simulink model "vsi_spwm"  (R2018a)
settings: Solver=FixedStepDiscrete  StartTime=0.0  StopTime=2/cfg.fl  FixedStep=cfg.fpga.ts  RelTol=1e-3
PreLoadFcn:
  | vsi_spwm_config;
InitFcn:
  | vsi_spwm_config;
undefined symbols (not defined in the file or in its folder): cfg
libraries: powerlib x18, hdlsllib x11, simulink x2
settings Model: DataTypeOverride=Off  Creator=CIDEI  LastModifiedBy=pcoss
settings DataIOCC: SaveOutput=off  SaveTime=off
settings OptimizationCC: BlockReduction=off  ConditionallyExecuteInputs=off  DefaultParameterBehavior=Inlined  LifeSpan=inf
settings DebuggingCC: AlgebraicLoopMsg=error  SingleTaskRateTransMsg=error  StrictBusMsg=ErrorOnBusTreatedAsVector  SFUnexpectedBacktrackingDiag=warning  SFNoUnconditionalDefaultTransitionDiag=warning  SFExecutionAtInitializationDiag=none
settings HardwareCC: ProdBitPerPointer=32  ProdBitPerSizeT=32  ProdBitPerPtrDiffT=32  ProdLargestAtomicFloat=None  ProdIntDivRoundTo=Undefined  ProdEndianess=Unspecified  ProdWordSize=32  ProdHWDeviceType=ASIC/FPGA->ASIC/FPGA  ProdEqTarget=off
settings CodeAppCC: StateflowObjectComments=on
settings GRTTargetCC: TargetLangStandard=C89/C90 (ANSI)
settings ConfigComp: CovMetricSettings=dw  CovHtmlReporting=on  CovSaveCumulativeToWorkspaceVar=on  CovSaveSingleToWorkspaceVar=on  CovExternalEMLEnable=off
settings SimscapeCC: SimscapeNormalizeSystem=off

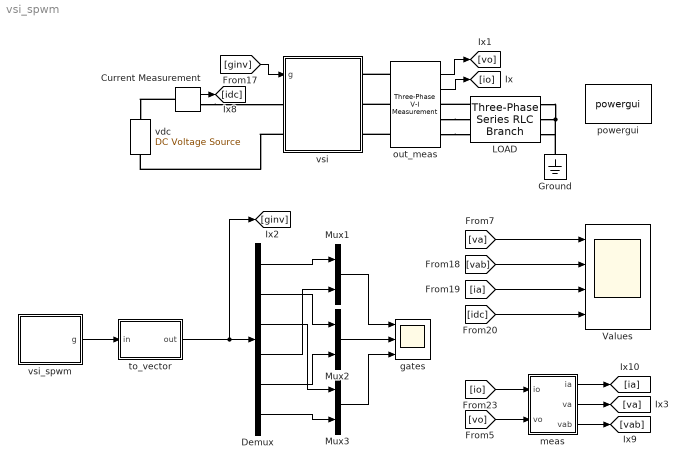
== system vsi_spwm ==
  Current Measurement : powerlib/Measurements/Current Measurement  PhasorSimulation=off  OutputType=Complex  PSBequivalent=0
  Demux : Demux  Outputs=6
  Ground : powerlib/Elements/Ground  LConnTagsString=a
  LOAD : powerlib/Elements/Three-Phase Series RLC Branch  LConnTagsString=A|B|C  RConnTagsString=A|B|C  BranchType=RL  Resistance=cfg.r  Inductance=cfg.l  Capacitance=1e-6  Measurements=None
  Mux1 : Mux  Inputs=2
  Mux2 : Mux  Inputs=2
  Mux3 : Mux  Inputs=2
  Values : Scope  NumInputPorts=4
  gates : Scope  NumInputPorts=3
  meas : Subsystem
  out_meas : powerlib/Measurements/Three-Phase V-I Measurement  VoltageMeasurement=phase-to-ground  SetLabelV=off  LabelV=Vabc  Vpu=off  VpuLL=off  CurrentMeasurement=yes  SetLabelI=off  LabelI=Iabc  Ipu=off  Pbase=100e6  Vbase=500e3  OutputType=Complex  PhasorSimulation=off  PSBequivalent=0
  powergui : powerlib/powergui  Priority=1  SimulationMode=Discrete  SampleTime=cfg.ts  frequency=60  Iterations=50  frequencyindice=0  Pbase=100e6  ErrMax=1e-4  UnitsV=kV  UnitsW=MW  buscounter=0  FunctionMessages=off  echomessages=off  EnableUseOfTLC=off  CurrentSourceSwitches=off  DisableSnubberDevices=off  DisableRonSwitches=off  DisableVfSwitches=off  DisplayEquations=off  SolverType=Backward Euler  Interpol=off  ExternalGateDelay=off  methode=off  Ts=0  x0status=blocks  SPID=off  SwTol=0  HookPort=off  RestoreLinks=warning  ResistiveCurrentMeasurement=off  Frange=[0:2:500]  Ylog=off  Xlog=on  ShowGrid=off  save=off  variable=ZData  structure=one_mod_model  ZoomFFT=off  StartTime=0.12  cycles=1  DisplayStyle=1  fundamental=50  FreqAxis=off  MaxFrequency=1000  frequencyindicesteady=1  RmsSteady=1  display=off
  to_vector : Subsystem
  vdc : powerlib/Electrical Sources/DC Voltage Source  Amplitude=cfg.vdc  Measurements=None
  vsi : Subsystem
  vsi_spwm : Subsystem
  wires:
  Mux2/1 -> gates/2
  Mux1/1 -> gates/1
  Mux3/1 -> gates/3
  Demux/4 -> Mux1/2
  Demux/5 -> Mux2/2
  Demux/6 -> Mux3/2
  out_meas/2 -> [io]
  out_meas/1 -> [vo]
  Current Measurement/1 -> [idc]
  [ginv] -> vsi/1(g)
  vsi_spwm/1(g) -> to_vector/1(in)
  Demux/1 -> Mux1/1
  Demux/2 -> Mux2/1
  Demux/3 -> Mux3/1
  [vab] -> Values/2
  [ia] -> Values/3
  [idc] -> Values/4
  [va] -> Values/1
  [io] -> meas/1(io)
  [vo] -> meas/2(vo)
  meas/1(ia) -> [ia]
  meas/3(vab) -> [vab]
  to_vector/1(out) -> [ginv], Demux/1
  meas/2(va) -> [va]
  connections:
  LOAD/RConn2 -- LOAD/RConn1 -- Ground/LConn1 -- LOAD/RConn3
  LOAD/LConn1 -- out_meas/RConn1
  Current Measurement/RConn1 -- vsi/LConn1
  out_meas/LConn2 -- vsi/RConn2
  out_meas/RConn3 -- LOAD/LConn3
  out_meas/RConn2 -- LOAD/LConn2
  out_meas/LConn1 -- vsi/RConn1
  out_meas/LConn3 -- vsi/RConn3
  Current Measurement/LConn1 -- vdc/RConn1
  vsi/LConn2 -- vdc/LConn1

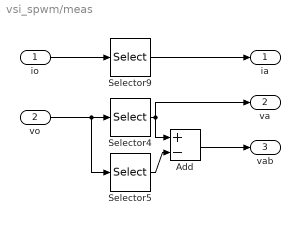
== system vsi_spwm/meas ==
  io : Inport
  vo : Inport  Port=2
  Add : Sum  Inputs=+-
  Selector4 : Selector  InputPortWidth=3  IndexOptions=Index vector (dialog)  Indices=1  OutputSizes=1
  Selector5 : Selector  InputPortWidth=3  IndexOptions=Index vector (dialog)  Indices=2  OutputSizes=1
  Selector9 : Selector  InputPortWidth=3  IndexOptions=Index vector (dialog)  Indices=1  OutputSizes=1
  ia : Outport
  va : Outport  Port=2
  vab : Outport  Port=3
  wires:
  vo/1 -> Selector5/1, Selector4/1
  Selector4/1 -> va/1, Add/1
  Selector5/1 -> Add/2
  Add/1 -> vab/1
  Selector9/1 -> ia/1
  io/1 -> Selector9/1

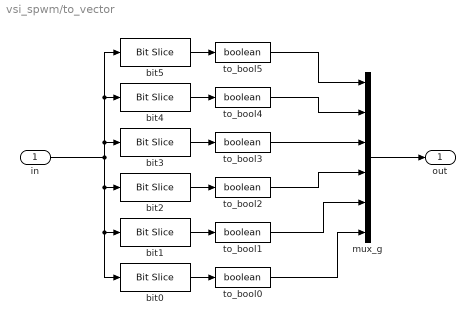
== system vsi_spwm/to_vector ==
  in : Inport
  bit0 : hdlsllib/Logic and Bit Operations/Bit Slice  lidx=0  ridx=0
  bit1 : hdlsllib/Logic and Bit Operations/Bit Slice  lidx=1  ridx=1
  bit2 : hdlsllib/Logic and Bit Operations/Bit Slice  lidx=2  ridx=2
  bit3 : hdlsllib/Logic and Bit Operations/Bit Slice  lidx=3  ridx=3
  bit4 : hdlsllib/Logic and Bit Operations/Bit Slice  lidx=4  ridx=4
  bit5 : hdlsllib/Logic and Bit Operations/Bit Slice  lidx=5  ridx=5
  mux_g : Mux  Inputs=6
  to_bool{0..5} (6 alike) : DataTypeConversion  OutDataTypeStr=boolean
  out : Outport
  wires:
  to_bool0/1 -> mux_g/6
  to_bool2/1 -> mux_g/4
  to_bool3/1 -> mux_g/3
  bit4/1 -> to_bool4/1
  bit5/1 -> to_bool5/1
  bit3/1 -> to_bool3/1
  bit2/1 -> to_bool2/1
  mux_g/1 -> out/1
  to_bool5/1 -> mux_g/1
  to_bool4/1 -> mux_g/2
  bit1/1 -> to_bool1/1
  to_bool1/1 -> mux_g/5
  in/1 -> bit5/1, bit4/1, bit3/1, bit2/1, bit1/1, bit0/1
  bit0/1 -> to_bool0/1

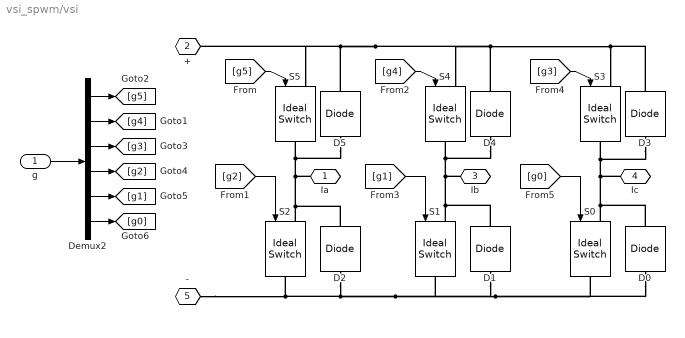
== system vsi_spwm/vsi ==
  g : Inport
  D{0..5} (6 alike) : powerlib/Power Electronics/Diode  Ron=cfg.diode.Ron  Lon=0  Vf=0  IC=0  UseSnubber=off  Rs=cfg.diode.snubber_Rs  Cs=cfg.diode.snubber_Cs  Measurements=off
  Demux2 : Demux  Outputs=6
  S{0..5} (6 alike) : powerlib/Power Electronics/Ideal Switch  Ron=cfg.switch.Ron  Lon=0  IC=0  Rs=cfg.switch.snubber_Rs  Cs=cfg.switch.snubber_Cs  Measurements=off
  Ia : PMIOPort  Side=Right
  + : PMIOPort  Port=2  Side=Left
  Ib : PMIOPort  Port=3  Side=Right
  Ic : PMIOPort  Port=4  Side=Right
  - : PMIOPort  Port=5  Side=Left
  wires:
  Demux2/1 -> [g5]
  Demux2/4 -> [g2]
  g/1 -> Demux2/1
  [g2] -> S2/1
  [g4] -> S4/1
  [g1] -> S1/1
  Demux2/5 -> [g1]
  [g3] -> S3/1
  [g0] -> S0/1
  Demux2/6 -> [g0]
  Demux2/3 -> [g3]
  Demux2/2 -> [g4]
  [g5] -> S5/1
  connections:
  S2/LConn1 -- D2/RConn1 -- D5/LConn1 -- S5/RConn1 -- Ia/RConn1
  S1/LConn1 -- D1/RConn1 -- D4/LConn1 -- S4/RConn1 -- Ib/RConn1
  S0/LConn1 -- D0/RConn1 -- D3/LConn1 -- S3/RConn1 -- Ic/RConn1
  S4/LConn1 -- D5/RConn1 -- S5/LConn1 -- +/RConn1 -- D3/RConn1 -- S3/LConn1 -- D4/RConn1
  -/RConn1 -- D1/LConn1 -- D0/LConn1 -- S0/RConn1 -- S1/RConn1 -- D2/LConn1 -- S2/RConn1

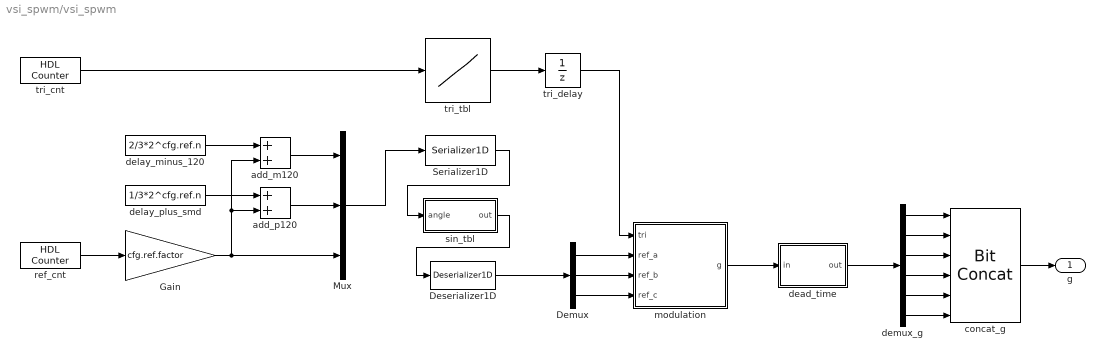
== system vsi_spwm/vsi_spwm ==
  Demux : Demux  Outputs=3
  Deserializer1D : hdlsllib/HDL Operations/Deserializer1D  Ratio=3  IdleCycles=0  InitialCondition=0  startIn=off  validIn=off  validOut=off  inputDataDimensions=-1  inputSampleTime=-1  inputSignalType=auto
      settings: SourceProductName=HDL Coder  SourceProductBaseCode=HD
  Gain : Gain  Gain=cfg.ref.factor  OutDataTypeStr=fixdt(0,cfg.ref.n,0)
  Mux : Mux  Inputs=3
  Serializer1D : hdlsllib/HDL Operations/Serializer1D  Ratio=3  IdleCycles=0  validIn=off  startOut=off  validOut=off  inputDataDimensions=-1  inputSampleTime=-1  inputSignalType=auto
      settings: SourceProductName=HDL Coder  SourceProductBaseCode=HD
  add_m120 : Sum  OutDataTypeStr=Inherit: Same as accumulator
  add_p120 : Sum  OutDataTypeStr=Inherit: Same as accumulator
  concat_g : hdlsllib/Logic and Bit Operations/Bit Concat  numInputs=6
      settings: SourceProductName=HDL Coder  SourceProductBaseCode=HD
  dead_time : Subsystem
  delay_minus_120 : Constant  Value=2/3*2^cfg.ref.n  OutDataTypeStr=fixdt(0,cfg.ref.n,0)  SampleTime=-1
  delay_plus_smd : Constant  Value=1/3*2^cfg.ref.n  OutDataTypeStr=fixdt(0,cfg.ref.n,0)  SampleTime=-1
  demux_g : Demux  Outputs=6
  modulation : Subsystem
  ref_cnt : hdlsllib/Sources/HDL Counter  CountType=Count limited  CountInit=0  CountStep=1  CountMax=1/cfg.fl/cfg.ts  CountFromType=Initial value  CountFrom=0  CountResetPort=off  CountLoadPort=off  CountEnbPort=off  CountDirPort=off  CountDataType=Unsigned  CountWordLen=ceil(log2(1/cfg.fl/cfg.ts))  CountFracLen=0  CountSampTime=cfg.ts
      settings: SourceProductBaseCode=HD
  sin_tbl : Subsystem
  tri_cnt : hdlsllib/Sources/HDL Counter  CountType=Count limited  CountInit=0  CountStep=1  CountMax=length(cfg.tri.data)-1  CountFromType=Initial value  CountFrom=0  CountResetPort=off  CountLoadPort=off  CountEnbPort=off  CountDirPort=off  CountDataType=Unsigned  CountWordLen=cfg.tri.n  CountFracLen=0  CountSampTime=cfg.ts
      settings: SourceProductBaseCode=HD
  tri_delay : UnitDelay  SampleTime=-1
  tri_tbl : Lookup_n-D  NumberOfTableDimensions=1  BreakpointsForDimension1=[0:length(cfg.tri.data)-1]  BreakpointsForDimension1FirstPoint=10  BreakpointsForDimension2FirstPoint=10  BreakpointsForDimension1Spacing=12  BreakpointsForDimension2Spacing=12  IndexSearchMethod=Evenly spaced points  Table=cfg.tri.data  InterpMethod=Flat  DiagnosticForOutOfRangeInput=Error  InternalRulePriority=Speed  OutDataTypeStr=fixdt(1,cfg.tri.out_n,0)  RndMeth=Simplest  InputSameDT=on
  g : Outport
  wires:
  Gain/1 -> add_p120/2, add_m120/2, Mux/3
  delay_plus_smd/1 -> add_p120/1
  tri_delay/1 -> modulation/1(tri)
  tri_tbl/1 -> tri_delay/1
  delay_minus_120/1 -> add_m120/1
  ref_cnt/1 -> Gain/1
  modulation/1(g) -> dead_time/1(in)
  add_m120/1 -> Mux/1
  add_p120/1 -> Mux/2
  Demux/2 -> modulation/3(ref_b)
  Demux/3 -> modulation/4(ref_c)
  Deserializer1D/1 -> Demux/1
  sin_tbl/1(out) -> Deserializer1D/1
  Serializer1D/1 -> sin_tbl/1(angle)
  Mux/1 -> Serializer1D/1
  Demux/1 -> modulation/2(ref_a)
  tri_cnt/1 -> tri_tbl/1
  demux_g/1 -> concat_g/1
  demux_g/2 -> concat_g/2
  demux_g/3 -> concat_g/3
  demux_g/4 -> concat_g/4
  demux_g/5 -> concat_g/5
  demux_g/6 -> concat_g/6
  dead_time/1(out) -> demux_g/1
  concat_g/1 -> g/1

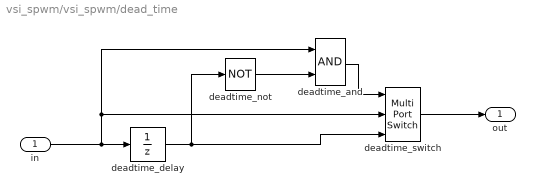
== system vsi_spwm/vsi_spwm/dead_time ==
  in : Inport
  deadtime_and : Logic  AllPortsSameDT=off  OutDataTypeStr=boolean
  deadtime_delay : UnitDelay  SampleTime=-1
  deadtime_not : Logic  Operator=NOT  AllPortsSameDT=off  OutDataTypeStr=boolean
  deadtime_switch : MultiPortSwitch  DataPortOrder=Zero-based contiguous  Inputs=2  zeroidx=on
  out : Outport
  wires:
  deadtime_not/1 -> deadtime_and/2
  deadtime_switch/1 -> out/1
  in/1 -> deadtime_delay/1, deadtime_switch/2, deadtime_and/1
  deadtime_delay/1 -> deadtime_switch/3, deadtime_not/1
  deadtime_and/1 -> deadtime_switch/1

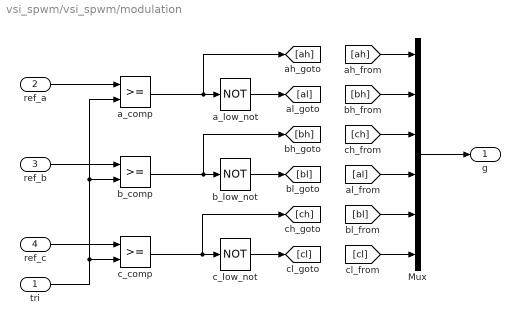
== system vsi_spwm/vsi_spwm/modulation ==
  tri : Inport
  ref_a : Inport  Port=2
  ref_b : Inport  Port=3
  ref_c : Inport  Port=4
  Mux : Mux  Inputs=6
  a_comp : RelationalOperator  OutDataTypeStr=boolean  RndMeth=Nearest
  a_low_not : Logic  Operator=NOT  AllPortsSameDT=off  OutDataTypeStr=boolean
  b_comp : RelationalOperator  OutDataTypeStr=boolean  RndMeth=Nearest
  b_low_not : Logic  Operator=NOT  AllPortsSameDT=off  OutDataTypeStr=boolean
  c_comp : RelationalOperator  OutDataTypeStr=boolean  RndMeth=Nearest
  c_low_not : Logic  Operator=NOT  AllPortsSameDT=off  OutDataTypeStr=boolean
  g : Outport
  wires:
  c_comp/1 -> [ch], c_low_not/1
  a_comp/1 -> [ah], a_low_not/1
  b_comp/1 -> [bh], b_low_not/1
  tri/1 -> a_comp/2, b_comp/2, c_comp/2
  ref_a/1 -> a_comp/1
  ref_b/1 -> b_comp/1
  ref_c/1 -> c_comp/1
  Mux/1 -> g/1
  c_low_not/1 -> [cl]
  b_low_not/1 -> [bl]
  a_low_not/1 -> [al]
  [cl] -> Mux/6
  [bl] -> Mux/5
  [al] -> Mux/4
  [ch] -> Mux/3
  [bh] -> Mux/2
  [ah] -> Mux/1

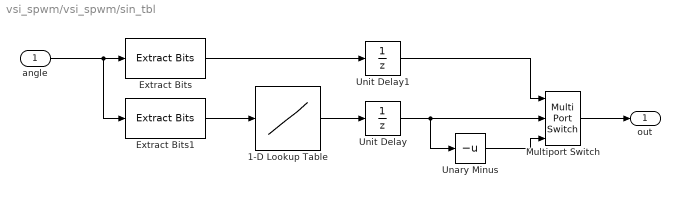
== system vsi_spwm/vsi_spwm/sin_tbl ==
  angle : Inport
  1-D Lookup Table : Lookup_n-D  NumberOfTableDimensions=1  BreakpointsForDimension1=[0:length(cfg.ref.data)-1]  BreakpointsForDimension1FirstPoint=10  BreakpointsForDimension2FirstPoint=10  BreakpointsForDimension1Spacing=12  BreakpointsForDimension2Spacing=12  IndexSearchMethod=Evenly spaced points  Table=cfg.ref.data  InterpMethod=Flat  DiagnosticForOutOfRangeInput=Error  InternalRulePriority=Speed  OutDataTypeStr=fixdt(1,cfg.ref.out_n,cfg.ref.out_n_bp)  RndMeth=Simplest  InputSameDT=on
  Extract Bits : simulink/Logic and Bit Operations/Extract Bits  bitsToExtract=Range starting with most significant bit  numBits=1  bitIdxRange=[0 7]  outScalingMode=Treat bit field as an integer
      settings: SourceProductName=Simulink
  Extract Bits1 : simulink/Logic and Bit Operations/Extract Bits  bitsToExtract=Range ending with least significant bit  numBits=cfg.ref.n-1  bitIdxRange=[0 7]  outScalingMode=Preserve fixed-point scaling
      settings: SourceProductName=Simulink
  Multiport Switch : MultiPortSwitch  DataPortOrder=Zero-based contiguous  Inputs=2  zeroidx=on
  Unary Minus : UnaryMinus
  Unit Delay : UnitDelay  SampleTime=-1
  Unit Delay1 : UnitDelay  SampleTime=-1
  out : Outport
  wires:
  Unit Delay1/1 -> Multiport Switch/1
  Extract Bits1/1 -> 1-D Lookup Table/1
  Extract Bits/1 -> Unit Delay1/1
  Multiport Switch/1 -> out/1
  angle/1 -> Extract Bits1/1, Extract Bits/1
  1-D Lookup Table/1 -> Unit Delay/1
  Unary Minus/1 -> Multiport Switch/3
  Unit Delay/1 -> Multiport Switch/2, Unary Minus/1
